simulink model "Ejercicio9_13_02_17"  (R2013a)
settings: Solver=ode45  StartTime=0.0  StopTime=20  RelTol=1e-3
settings Model: Creator=Miguel  LastModifiedBy=Miguel

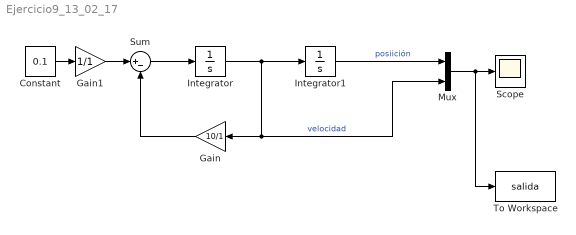
== system Ejercicio9_13_02_17 ==
  Constant : Constant  Value=0.1
  Gain : Gain  Gain=10/1
  Gain1 : Gain  Gain=1/1
  Integrator : Integrator  InitialCondition=-1
  Integrator1 : Integrator
  Mux : Mux  Inputs=2
  Scope : Scope
      settings: ShowLegends=on
  Sum : Sum  Inputs=|+-
  To Workspace : ToWorkspace  VariableName=salida  SampleTime=-1
  wires:
  Constant/1 -> Gain1/1
  Sum/1 -> Integrator/1
  Integrator/1 -> Gain/1, Mux/2, Integrator1/1  "velocidad"
  Integrator1/1 -> Mux/1  "posiición"
  Mux/1 -> To Workspace/1, Scope/1
  Gain1/1 -> Sum/1
  Gain/1 -> Sum/2
